simulink subsystem "Batteri"  (R2020b)
settings: Solver=VariableStepAuto  StartTime=0.0  StopTime=10.0  RelTol=1e-3
libraries: fl_lib x82, ee_lib x28, nesl_utility x3
(part 2 of 2)

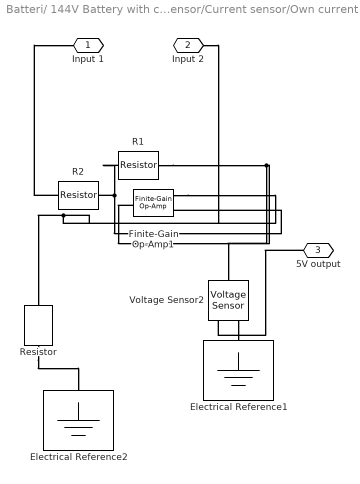
== system Batteri/ 144V Battery with current sensor/Current sensor/Own current sensor ==
  Electrical Reference1 : fl_lib/Electrical/Electrical Elements/Electrical Reference
  Electrical Reference2 : fl_lib/Electrical/Electrical Elements/Electrical Reference
  Finite-Gain Op-Amp1 : ee_lib/Integrated Circuits/Finite-Gain Op-Amp  A=1000  Rin=1e6 Ohm  Rout=0 Ohm  Vmin=0 V  Vmax=5 V  noise_mode=0  v_noise=30e-9 V/Hz^0.50000  noise_prm=1  i_noise=0.5e-12 A/Hz^0.50000  ip_noise=0.5e-12 A/Hz^0.50000  in_noise=0.5e-12 A/Hz^0.50000  sample_time=1e-3 s  repeatability=1  auto_seed_v=734023807  auto_seed_ip=1714822877  auto_seed_in=2996382080  user_seed_v=0  user_seed_ip=0  user_seed_in=0
      settings: SourceProductBaseCode=PS  InternalSimscapePortConfiguration="{\"Bottom\":[],\"Left\":[{\"id\":\"p\",\"label\":\"+\",\"type\":\"foundation.electrical.electrical\"},{\"id\":\"n\",\"label\":\"-\",\"type\":\"foundation.electrical.electrical\"}],\"Right\":[{\"id\":\"out\",\"label\":\"\",\"type\":\"foundation.electrical.electrical\"}],\"Top\":[]}"
  R1 : fl_lib/Electrical/Electrical Elements/Resistor  R=16 Ohm  i_specify=off  i_priority=None  i=0 A  i_nominal_specify=off  i_nominal_unit=A  i_nominal_value=1  v_specify=off  v_priority=None  v=0 V  v_nominal_specify=off  v_nominal_unit=V  v_nominal_value=1
  R2 : fl_lib/Electrical/Electrical Elements/Resistor  R=1 Ohm  i_specify=off  i_priority=None  i=0 A  i_nominal_specify=off  i_nominal_unit=A  i_nominal_value=1  v_specify=off  v_priority=None  v=0 V  v_nominal_specify=off  v_nominal_unit=V  v_nominal_value=1
  Resistor : fl_lib/Electrical/Electrical Elements/Resistor  R=1 Ohm  i_specify=off  i_priority=None  i=0 A  i_nominal_specify=off  i_nominal_unit=A  i_nominal_value=1  v_specify=off  v_priority=None  v=0 V  v_nominal_specify=off  v_nominal_unit=V  v_nominal_value=1
  Voltage Sensor2 : fl_lib/Electrical/Electrical Sensors/Voltage Sensor
  Input 1 : PMIOPort  Side=Left
  Input 2 : PMIOPort  Port=2  Side=Left
  5V output : PMIOPort  Port=3  Side=Right
  connections:
  5V output/RConn1 -- Voltage Sensor2/RConn1
  Voltage Sensor2/RConn2 -- Electrical Reference1/LConn1
  Finite-Gain Op-Amp1/LConn1 -- Resistor/LConn1 -- Input 2/RConn1
  Finite-Gain Op-Amp1/LConn2 -- R2/RConn1 -- R1/LConn1
  R1/RConn1 -- Finite-Gain Op-Amp1/RConn1 -- Voltage Sensor2/LConn1
  R2/LConn1 -- Input 1/RConn1
  Resistor/RConn1 -- Electrical Reference2/LConn1

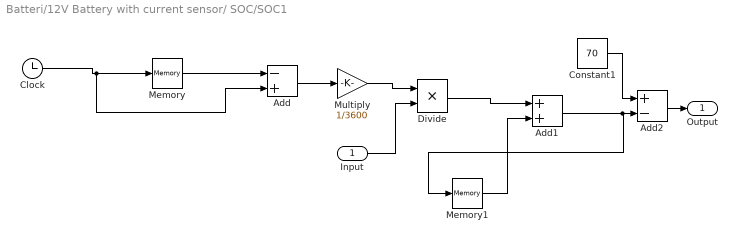
== system Batteri/12V Battery with current sensor/ SOC/SOC1 ==
  Input : Inport
  Add : Sum  Inputs=-+
  Add1 : Sum
  Add2 : Sum  Inputs=+-
  Clock : Clock
  Constant1 : Constant  Value=70  SampleTime=-1
  Divide : Product  Inputs=**
  Memory : Memory
  Memory1 : Memory
  Multiply : Gain  Gain=1/3600
  Output : Outport
  wires:
  Clock/1 -> Add/2, Memory/1
  Memory/1 -> Add/1
  Add/1 -> Multiply/1
  Memory1/1 -> Add1/2
  Add1/1 -> Memory1/1, Add2/2
  Input/1 -> Divide/2
  Multiply/1 -> Divide/1
  Divide/1 -> Add1/1
  Add2/1 -> Output/1
  Constant1/1 -> Add2/1

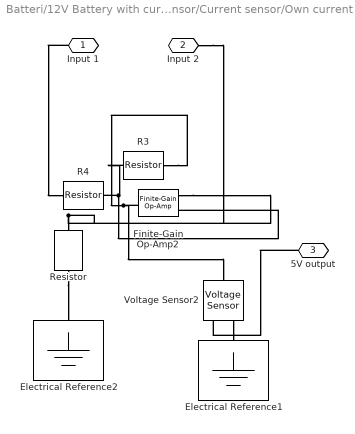
== system Batteri/12V Battery with current sensor/Current sensor/Own current sensor ==
  Electrical Reference1 : fl_lib/Electrical/Electrical Elements/Electrical Reference
  Electrical Reference2 : fl_lib/Electrical/Electrical Elements/Electrical Reference
  Finite-Gain Op-Amp2 : ee_lib/Integrated Circuits/Finite-Gain Op-Amp  A=1000  Rin=1e6 Ohm  Rout=0 Ohm  Vmin=0 V  Vmax=5 V  noise_mode=0  v_noise=30e-9 V/Hz^0.50000  noise_prm=1  i_noise=0.5e-12 A/Hz^0.50000  ip_noise=0.5e-12 A/Hz^0.50000  in_noise=0.5e-12 A/Hz^0.50000  sample_time=1e-3 s  repeatability=1  auto_seed_v=874783637  auto_seed_ip=2861850476  auto_seed_in=1902954364  user_seed_v=0  user_seed_ip=0  user_seed_in=0
      settings: SourceProductBaseCode=PS  InternalSimscapePortConfiguration="{\"Bottom\":[],\"Left\":[{\"id\":\"p\",\"label\":\"+\",\"type\":\"foundation.electrical.electrical\"},{\"id\":\"n\",\"label\":\"-\",\"type\":\"foundation.electrical.electrical\"}],\"Right\":[{\"id\":\"out\",\"label\":\"\",\"type\":\"foundation.electrical.electrical\"}],\"Top\":[]}"
  R3 : fl_lib/Electrical/Electrical Elements/Resistor  R=300 Ohm  i_specify=off  i_priority=None  i=0 A  i_nominal_specify=off  i_nominal_unit=A  i_nominal_value=1  v_specify=off  v_priority=None  v=0 V  v_nominal_specify=off  v_nominal_unit=V  v_nominal_value=1
  R4 : fl_lib/Electrical/Electrical Elements/Resistor  R=1 Ohm  i_specify=off  i_priority=None  i=0 A  i_nominal_specify=off  i_nominal_unit=A  i_nominal_value=1  v_specify=off  v_priority=None  v=0 V  v_nominal_specify=off  v_nominal_unit=V  v_nominal_value=1
  Resistor : fl_lib/Electrical/Electrical Elements/Resistor  R=1 Ohm  i_specify=off  i_priority=None  i=0 A  i_nominal_specify=off  i_nominal_unit=A  i_nominal_value=1  v_specify=off  v_priority=None  v=0 V  v_nominal_specify=off  v_nominal_unit=V  v_nominal_value=1
  Voltage Sensor2 : fl_lib/Electrical/Electrical Sensors/Voltage Sensor
  Input 1 : PMIOPort  Side=Left
  Input 2 : PMIOPort  Port=2  Side=Left
  5V output : PMIOPort  Port=3  Side=Right
  connections:
  5V output/RConn1 -- Voltage Sensor2/RConn1
  Voltage Sensor2/RConn2 -- Electrical Reference1/LConn1
  R3/LConn1 -- Finite-Gain Op-Amp2/LConn2 -- R4/RConn1
  Finite-Gain Op-Amp2/LConn1 -- Resistor/LConn1 -- Input 2/RConn1
  R3/RConn1 -- Finite-Gain Op-Amp2/RConn1 -- Voltage Sensor2/LConn1
  Input 1/RConn1 -- R4/LConn1
  Resistor/RConn1 -- Electrical Reference2/LConn1
